simulink model "ITAEmodPID"  (R2024b)
settings: Solver=ode5  StartTime=0.0  StopTime=2  FixedStep=1e-5  RelTol=1e-3
values from neighbouring files (symbols this model uses):
  J = out.J_ITAE_PI.Data    [ITAE_PI.m]    (also in ITAE_PID.m = out.J_ITAE_PID.Data)
undefined symbols (not defined in the file or in its folder): A, B, C, D, g, ke, Kp, L, N, R, rho, Td, Ti
settings Model: Creator=Lukáš Zezula  LastModifiedBy=tomse
settings RTWCC: GPUComputeCapability=3.5

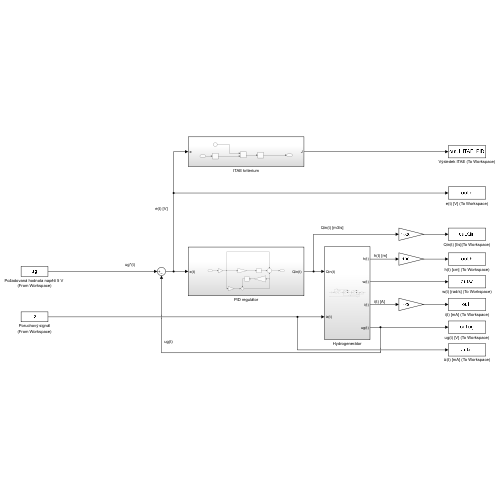
[thumbnail: Simulink's stored preview of the top-level diagram]
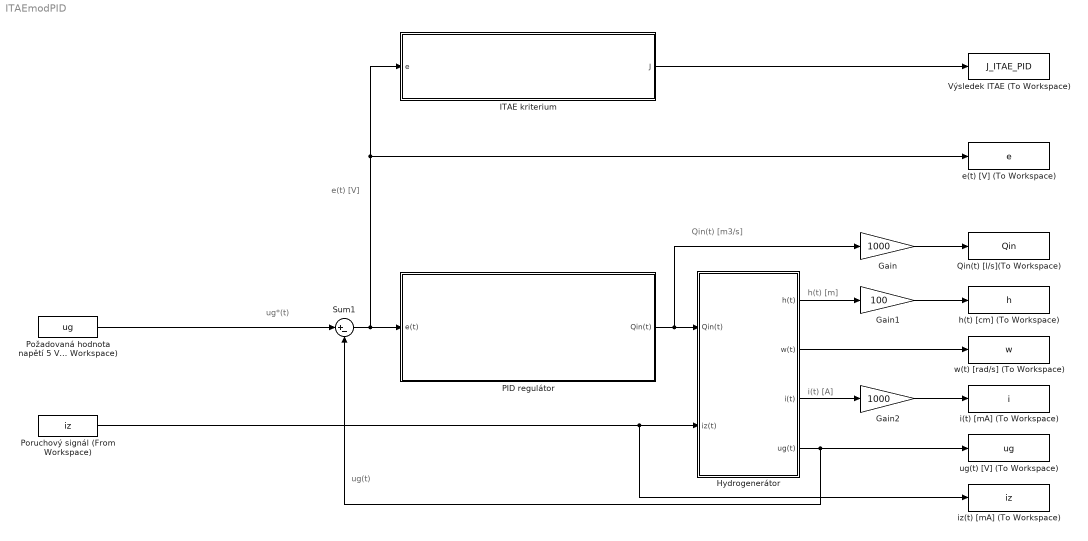
== system ITAEmodPID ==
  note: ug(t)
  note: ug*(t)
  note: Qin(t) [m3/s]
  note: h(t) [m]
  note: i(t) [A]
  note: e(t) [V]
  Gain : Gain  Gain=1000
  Gain1 : Gain  Gain=100
  Gain2 : Gain  Gain=1000
  Hydrogenerátor : Subsystem
  ITAE kriterium : Subsystem
  PID regulátor : Subsystem
  Poruchový signál (From Workspace) : FromWorkspace  VariableName=iz
  Požadovaná hodnota napětí 5 V (From Workspace) : FromWorkspace  VariableName=ug
  Qin(t) [l/s](To Workspace) : ToWorkspace  VariableName=Qin  SaveFormat=Timeseries  SampleTime=-1
  Sum1 : Sum  Inputs=|+-
  Výsledek ITAE (To Workspace) : ToWorkspace  VariableName=J_ITAE_PID  SaveFormat=Timeseries  SampleTime=-1
      settings: MaxDataPoints=1
  e(t) [V] (To Workspace) : ToWorkspace  VariableName=e  SaveFormat=Timeseries  SampleTime=-1
  h(t) [cm] (To Workspace) : ToWorkspace  VariableName=h  SaveFormat=Timeseries  SampleTime=-1
  i(t) [mA] (To Workspace) : ToWorkspace  VariableName=i  SaveFormat=Timeseries  SampleTime=-1
  iz(t) [mA] (To Workspace) : ToWorkspace  VariableName=iz  SaveFormat=Timeseries  SampleTime=-1
  ug(t) [V] (To Workspace) : ToWorkspace  VariableName=ug  SaveFormat=Timeseries  SampleTime=-1
  w(t) [rad/s] (To Workspace) : ToWorkspace  VariableName=w  SaveFormat=Timeseries  SampleTime=-1
  wires:
  Gain2/1 -> i(t) [mA] (To Workspace)/1
  Hydrogenerátor/4(ug(t)) -> Sum1/2, ug(t) [V] (To Workspace)/1
  Požadovaná hodnota napětí 5 V (From Workspace)/1 -> Sum1/1
  Gain1/1 -> h(t) [cm] (To Workspace)/1
  Gain/1 -> Qin(t) [l/s](To Workspace)/1
  Hydrogenerátor/1(h(t)) -> Gain1/1
  Hydrogenerátor/2(w(t)) -> w(t) [rad/s] (To Workspace)/1
  Poruchový signál (From Workspace)/1 -> iz(t) [mA] (To Workspace)/1, Hydrogenerátor/2(iz(t))
  ITAE kriterium/1(J) -> Výsledek ITAE (To Workspace)/1
  Hydrogenerátor/3(i(t)) -> Gain2/1
  Sum1/1 -> ITAE kriterium/1(e), e(t) [V] (To Workspace)/1, PID regulátor/1(e(t))
  PID regulátor/1("Qin(t) ") -> Gain/1, Hydrogenerátor/1(Qin(t))

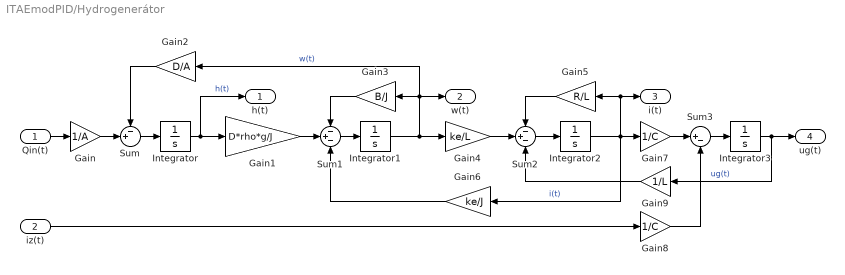
== system ITAEmodPID/Hydrogenerátor ==
  Qin(t) : Inport
  iz(t) : Inport  Port=2
  Gain : Gain  Gain=1/A
  Gain1 : Gain  Gain=D*rho*g/J
  Gain2 : Gain  Gain=D/A
  Gain3 : Gain  Gain=B/J
  Gain4 : Gain  Gain=ke/L
  Gain5 : Gain  Gain=R/L
  Gain6 : Gain  Gain=ke/J
  Gain7 : Gain  Gain=1/C
  Gain8 : Gain  Gain=1/C
  Gain9 : Gain  Gain=1/L
  Integrator{,1..3} (4 alike) : Integrator
  Sum : Sum  Inputs=-+|
  Sum1 : Sum  Inputs=-+-
  Sum2 : Sum  Inputs=-+-
  Sum3 : Sum  Inputs=|+-
  h(t) : Outport
  w(t) : Outport  Port=2
  i(t) : Outport  Port=3
  ug(t) : Outport  Port=4
  wires:
  Qin(t)/1 -> Gain/1
  Integrator/1 -> h(t)/1, Gain1/1  "h(t)"
  Sum/1 -> Integrator/1
  Gain1/1 -> Sum1/2
  Sum1/1 -> Integrator1/1
  Integrator1/1 -> Gain4/1, Gain2/1, Gain3/1, w(t)/1  "w(t)"
  Gain/1 -> Sum/2
  Gain2/1 -> Sum/1
  Gain3/1 -> Sum1/1
  Gain4/1 -> Sum2/2
  Sum2/1 -> Integrator2/1
  Gain5/1 -> Sum2/1
  Integrator2/1 -> Gain7/1, i(t)/1, Gain5/1, Gain6/1  "i(t)"
  Gain6/1 -> Sum1/3
  iz(t)/1 -> Gain8/1
  Gain7/1 -> Sum3/1
  Gain8/1 -> Sum3/2
  Sum3/1 -> Integrator3/1
  Integrator3/1 -> Gain9/1, ug(t)/1  "ug(t)"
  Gain9/1 -> Sum2/3

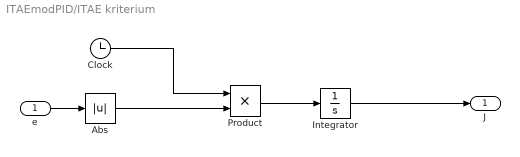
== system ITAEmodPID/ITAE kriterium ==
  e : Inport
  Abs : Abs  SaturateOnIntegerOverflow=off
  Clock : Clock
  Integrator : Integrator
  Product : Product
  J : Outport
  wires:
  e/1 -> Abs/1
  Product/1 -> Integrator/1
  Abs/1 -> Product/2
  Clock/1 -> Product/1
  Integrator/1 -> J/1

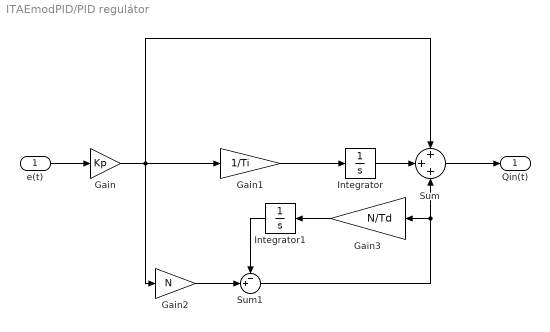
== system ITAEmodPID/PID regulátor ==
  e(t) : Inport
  Gain : Gain  Gain=Kp
  Gain1 : Gain  Gain=1/Ti
  Gain2 : Gain  Gain=N
  Gain3 : Gain  Gain=N/Td
  Integrator : Integrator
  Integrator1 : Integrator
  Sum : Sum  Inputs=+++
  Sum1 : Sum  Inputs=-+|
  "Qin(t) " : Outport
  wires:
  Integrator1/1 -> Sum1/1
  Gain3/1 -> Integrator1/1
  Sum1/1 -> Gain3/1, Sum/3
  Gain2/1 -> Sum1/2
  Integrator/1 -> Sum/2
  Gain1/1 -> Integrator/1
  Gain/1 -> Gain1/1, Sum/1, Gain2/1
  Sum/1 -> "Qin(t) "/1
  e(t)/1 -> Gain/1
